simulink model "Parameter_Estimation_Model"  (R2014b)
settings: Solver=ode45  StartTime=0.0  StopTime=10.0  RelTol=1e-3
undefined symbols (not defined in the file or in its folder): A1, A2, B1, B2, C1, C2, C3, C4
libraries: simulink x2
settings Model: Creator=z51  LastModifiedBy=z51

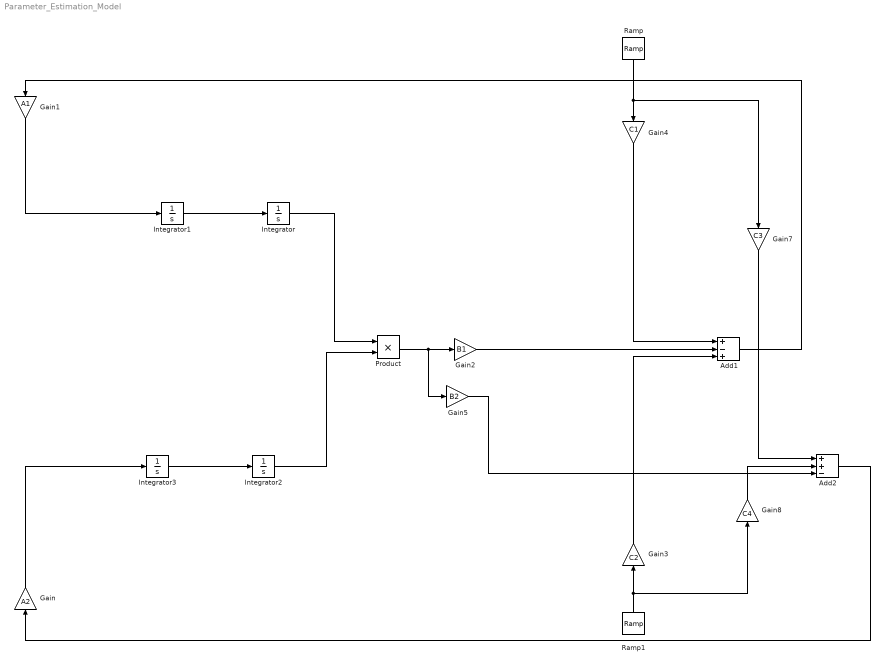
== system Parameter_Estimation_Model ==
  Add1 : Sum  Inputs=+-+
  Add2 : Sum  Inputs=++-
  Gain : Gain  Gain=A2
  Gain1 : Gain  Gain=A1
  Gain2 : Gain  Gain=B1
  Gain3 : Gain  Gain=C2
  Gain4 : Gain  Gain=C1
  Gain5 : Gain  Gain=B2
  Gain7 : Gain  Gain=C3
  Gain8 : Gain  Gain=C4
  Integrator{,1..3} (4 alike) : Integrator
  Product : Product
  Ramp : simulink/Sources/Ramp  slope=1  start=0  X0=0
  Ramp1 : simulink/Sources/Ramp  slope=1  start=0  X0=0
  wires:
  Integrator1/1 -> Integrator/1
  Integrator/1 -> Product/1
  Integrator3/1 -> Integrator2/1
  Integrator2/1 -> Product/2
  Gain/1 -> Integrator3/1
  Gain1/1 -> Integrator1/1
  Product/1 -> Gain5/1, Gain2/1
  Gain2/1 -> Add1/2
  Gain4/1 -> Add1/1
  Gain3/1 -> Add1/3
  Add1/1 -> Gain1/1
  Add2/1 -> Gain/1
  Gain5/1 -> Add2/3
  Gain7/1 -> Add2/1
  Gain8/1 -> Add2/2
  Ramp1/1 -> Gain8/1, Gain3/1
  Ramp/1 -> Gain7/1, Gain4/1
